simulink model "model01"  (R2023a)
settings: Solver=VariableStepAuto  StartTime=0.0  StopTime=0.04  RelTol=1e-3
libraries: spsSeriesRLCBranchLib x2, spsVoltageMeasurementLib x1, spsDCVoltageSourceLib x1, spsDiodeLib x1, spsIdealSwitchLib x1, spsStairGeneratorLib x1, sps_lib x1
settings Model: Creator=pc  LastModifiedBy=pc

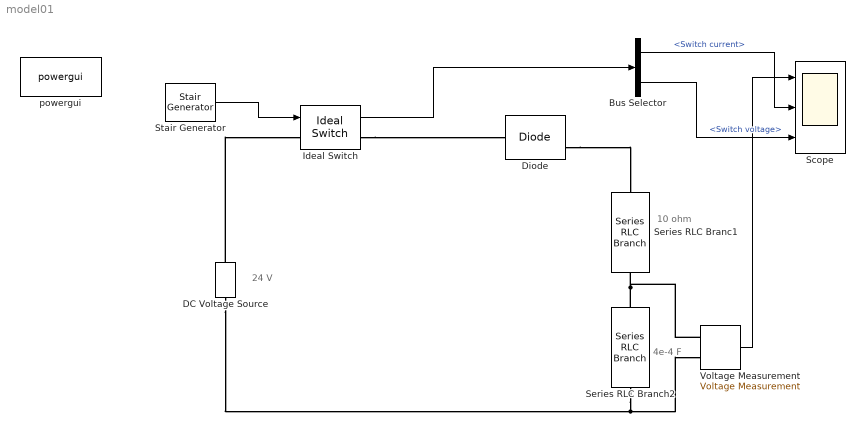
== system model01 ==
  note: 24 V
  note: 4e-4 F
  note: 10 ohm
  "                 Voltage Measurement" : spsVoltageMeasurementLib/Voltage Measurement  PhasorSimulation=off  OutputType=Complex  PSBequivalent=0
  Bus Selector : BusSelector  OutputSignals=Switch current,Switch voltage
  DC Voltage Source : spsDCVoltageSourceLib/DC Voltage Source  Amplitude=24  Measurements=None
  Diode : spsDiodeLib/Diode  Ron=0.001  Lon=0  Vf=0.8  IC=0  UseSnubber=0  Rs=500  Cs=250e-9  Measurements=on
  Ideal Switch : spsIdealSwitchLib/Ideal Switch  Ron=0.001  Lon=0  IC=0  Rs=1e5  Cs=inf  Measurements=on
  Scope : Scope  NumInputPorts=3
  Series RLC Branc1 : spsSeriesRLCBranchLib/Series RLC Branch  LConnTagsString=__new0  RConnTagsString=__new0  BranchType=R  Resistance=5  Inductance=1e-3  SetiL0=off  InitialCurrent=0  Capacitance=1e-6  Setx0=off  InitialVoltage=0  Measurements=None
  Series RLC Branch2 : spsSeriesRLCBranchLib/Series RLC Branch  LConnTagsString=__new0  RConnTagsString=__new0  BranchType=C  Resistance=1  Inductance=1e-3  SetiL0=off  InitialCurrent=0  Capacitance=4e-4  Setx0=off  InitialVoltage=0  Measurements=None
  Stair Generator : spsStairGeneratorLib/Stair Generator  t=[0, 1, 3, 3.5]  e=[1, -1, 2.5, 0]  Ts=0
  powergui : sps_lib/powergui  Priority=1  SimulationMode=Continuous  SampleTime=50e-6  frequency=60  Iterations=50  frequencyindice=0  Pbase=100e6  ErrMax=1e-4  UnitsV=kV  UnitsW=MW  buscounter=0  FunctionMessages=off  echomessages=off  EnableUseOfTLC=off  CurrentSourceSwitches=off  DisableSnubberDevices=off  DisableRonSwitches=off  DisableVfSwitches=off  DisplayEquations=off  AutomaticDiscreteSolvers=off  SolverType=Tustin/Backward Euler (TBE)  Interpol=off  ExternalGateDelay=off  methode=off  Ts=100  x0status=blocks  SPID=on  SwTol=0  HookPort=off  NonlinearTolerance=1e-4  nMaxIteration=100  ContinueOnMaxIteration=off  RestoreLinks=warning  ResistiveCurrentMeasurement=off  Frange=[0:2:500]  Ylog=off  Xlog=on  ShowGrid=off  save=off  variable=ZData  structure=0  ZoomFFT=off  StartTime=0.0  cycles=1  DisplayStyle=1  fundamental=60  FreqAxis=off  MaxFrequency=1000  frequencyindicesteady=1  RmsSteady=1  display=off
  wires:
  "                 Voltage Measurement"/1 -> Scope/1
  Bus Selector/1 -> Scope/2  "<Switch current>"
  Bus Selector/2 -> Scope/3  "<Switch voltage>"
  Stair Generator/1 -> Ideal Switch/1
  Ideal Switch/1 -> Bus Selector/1
  connections:
  DC Voltage Source/LConn1 -- Series RLC Branch2/RConn1 -- "                 Voltage Measurement"/LConn2
  "                 Voltage Measurement"/LConn1 -- Series RLC Branch2/LConn1 -- Series RLC Branc1/RConn1
  Diode/RConn1 -- Series RLC Branc1/LConn1
  Ideal Switch/RConn1 -- Diode/LConn1
  DC Voltage Source/RConn1 -- Ideal Switch/LConn1
